simulink model "sim8"  (R2015b)
settings: Solver=VariableStepAuto  StartTime=0.0  StopTime=10.0  RelTol=1e-3
values from neighbouring files (symbols this model uses):
  dy_inicial = 0    [Lab2.m]
  K = 10000    [Lab2.m]
  y_inicial = 1    [Lab2.m]
settings Model: Creator=Alice  LastModifiedBy=Alice

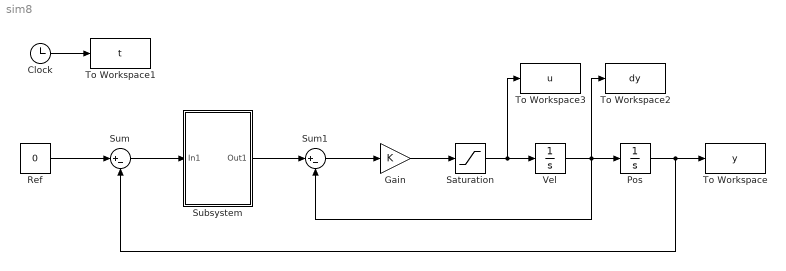
== system sim8 ==
  Clock : Clock
  Gain : Gain  Gain=K
  Pos : Integrator  InitialCondition=y_inicial
  Ref : Constant  Value=0
  Saturation : Saturate  UpperLimit=1  LowerLimit=-1
  Subsystem : Subsystem
  Sum : Sum  Inputs=|+-
  Sum1 : Sum  Inputs=|+-
  To Workspace : ToWorkspace  VariableName=y  SampleTime=0.1
  To Workspace1 : ToWorkspace  VariableName=t  SampleTime=0.1
  To Workspace2 : ToWorkspace  VariableName=dy  SampleTime=0.1
  To Workspace3 : ToWorkspace  VariableName=u  SampleTime=0.1
  Vel : Integrator  InitialCondition=dy_inicial
  wires:
  Ref/1 -> Sum/1
  Sum/1 -> Subsystem/1(In1)
  Subsystem/1(Out1) -> Sum1/1
  Sum1/1 -> Gain/1
  Gain/1 -> Saturation/1
  Saturation/1 -> To Workspace3/1, Vel/1
  Vel/1 -> To Workspace2/1, Sum1/2, Pos/1
  Pos/1 -> To Workspace/1, Sum/2
  Clock/1 -> To Workspace1/1

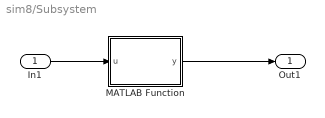
== system sim8/Subsystem ==
  In1 : Inport
  MATLAB Function : MATLAB Function  TreatAsAtomicUnit=on
  Out1 : Outport
  wires:
  In1/1 -> MATLAB Function/1(u)
  MATLAB Function/1(y) -> Out1/1

== matlab function sim8/Subsystem/MATLAB Function ==
  data: u input; y output
function y = fcn(u)

y=sign(u)*sqrt(2*abs(u));

end
